simulink model "IEEE34bus_v2019b_Phasor_PI_ZIPload"  (R2024a)
settings: Solver=ode4  StartTime=0.0  StopTime=60  FixedStep=Ts  MaxStep=1e-4  RelTol=1e-4
InitFcn:
  | a=1; % Loading Factor
  | Ts=0.1;% For Delay Blocks in Voltage Regulator Controls
  | % phase to sequence conversion of RXB matrices
  | c=1*exp(sqrt(-1)*(120*pi/180));
  | T=[1 1 1;1 c*c c;1 c c*c];
  | Tinv=1/3*[1 1 1;1 c c*c;1 c*c c];
  | 
  | % Simulation data for the IEEE 34 Node Test Feeder model
  | mi2km = 1.60934;%  miles to km conversion
  | ft2km = 0.0003048; % feet to km conversion
  | ms2F = 1*1e-6/(2*pi*60);% microsiemens to Farads conversion
  | 
  | %% Configuration 300 - series reactance - ohm/mile
  | R_300 = [1.3368 0.2101 0.2130;0.2101 1.3238 0.2066;0.2130 0.2066 1.3294];
  | X_300 = [1.3343 0.5779 0.5015;0.5779 1.3569 0.4591;0.5015 0.4591 1.3471];
  | % charging susceptance - microsiemens/mile
  | B_300 = [5.3350 -1.5313 -0.9943;-1.5313 5.0979 -0.6212;-0.9943 -0.6212 4.8880];
  | 
  | R_300 = R_300/mi2km;
  | Rseq=Tinv*R_300*T;
  | R1_300=Rseq(2,2);R0_300=Rseq(1,1);
  | 
  | L_300 = (X_300/(2*pi*60))/mi2km;
  | Lseq=Tinv*L_300*T;
  | L1_300=Lseq(2,2);L0_300=Lseq(1,1);
  | 
  | C_300 =(B_300*ms2F)/mi2km;
  | Cseq=Tinv*C_300*T;
  | C1_300=Cseq(2,2);C0_300=Cseq(1,1);
  | 
  | %% Configuration 301 - series reactance - ohm/mile
  | R_301 = [1.9300 0.2327 0.2359;0.2327 1.9157 0.2288;0.2359 0.2288 1.9219];
  | X_301 = [1.4115 0.6442 0.5691;0.6442 1.4281 0.5238;0.5691 0.5238 1.4209];
  | % charging susceptance - microsiemens/mile
  | B_301 = [5.1207 -1.4364 -0.9402;-1.4364 4.9055 -0.5951;-0.9402 -0.5951 4.7154];
  | 
  | R_301 = R_301/mi2km;
  | Rseq=Tinv*R_301*T;
  | R1_301=Rseq(2,2);R0_301=Rseq(1,1);
  | 
  | L_301 = (X_301/(2*pi*60))/mi2km;
  | Lseq=Tinv*L_301*T;
  | L1_301=Lseq(2,2);L0_301=Lseq(1,1);
  | 
  | C_301 =(B_301*ms2F)/mi2km;
  | Cseq=Tinv*C_301*T;
  | C1_301=Cseq(2,2);C0_301=Cseq(1,1);
  | 
  | %% Configuration 302 - series reactance - ohm/mile
  | R_302 = [2.7995 0 0;0 0 0;0 0 0];
  | X_302 = [1.4855 0 0;0 0 0;0 0 0];
  | % charging susceptance - microsiemens/mile
  | B_302 = [4.2251 0 0;0 0 0;0 0 0];
  | 
  | R_302 = R_302/mi2km;
  | Rseq=Tinv*R_302*T;
  | R1_302=Rseq(2,2);R0_302=Rseq(1,1);
  | 
  | L_302 = (X_302/(2*pi*60))/mi2km;
  | Lseq=Tinv*L_302*T;
  | ... (+41 lines)
undefined symbols (not defined in the file or in its folder): find_system, j, m1, m2, m3, Rcc1, Rcc2, Rcc3
libraries: spsSeriesRLCBranchLib x160, spsGroundLib x106, spsVoltageMeasurementLib x100, spsControlledCurrentSourceLib x94, spsPowerPhasorLib x57, spsThreePhaseVIMeasurementLib x37, spsThreePhasePISectionLineLib x20, spsCurrentMeasurementLib x12, spsOnDelayLib x12, spsPiSectionLineLib x11, spsControlledVoltageSourceLib x6, spsDiscreteVariableTimeDelayLib x6
(part 3 of 8)

== system IEEE34bus_v2019b_Phasor_PI_ZIPload/834 D PQ ==
  Controlled Current Source : spsControlledCurrentSourceLib/Controlled Current Source  Initialize=off  Source_Type=AC  Amplitude=0  Phase=0  Frequency=0  Measurements=None
  Controlled Current Source1 : spsControlledCurrentSourceLib/Controlled Current Source  Initialize=off  Source_Type=AC  Amplitude=0  Phase=0  Frequency=0  Measurements=None
  Controlled Current Source2 : spsControlledCurrentSourceLib/Controlled Current Source  Initialize=off  Source_Type=AC  Amplitude=0  Phase=0  Frequency=0  Measurements=None
  Demux1 : Demux  Outputs=3
  Embedded MATLAB Function2 : MATLAB Function  TreatAsAtomicUnit=on
  Gain4 : Gain  Gain=sqrt(2)
  Gain5 : Gain  Gain=1/sqrt(2)
  Memory3 : Memory
  Mux5 : Mux  Inputs=3
  Rc+jXc1 : spsSeriesRLCBranchLib/Series RLC Branch  LConnTagsString=__new0  RConnTagsString=__new0  BranchType=R  Resistance=1e6  Inductance=1.6 / (120*pi) * 2  SetiL0=off  InitialCurrent=0  Capacitance=1e-6  Setx0=off  InitialVoltage=0  Measurements=None
  Rc+jXc2 : spsSeriesRLCBranchLib/Series RLC Branch  LConnTagsString=__new0  RConnTagsString=__new0  BranchType=R  Resistance=1e6  Inductance=1.6 / (120*pi) * 2  SetiL0=off  InitialCurrent=0  Capacitance=1e-6  Setx0=off  InitialVoltage=0  Measurements=None
  Rc+jXc3 : spsSeriesRLCBranchLib/Series RLC Branch  LConnTagsString=__new0  RConnTagsString=__new0  BranchType=R  Resistance=1e6  Inductance=1.6 / (120*pi) * 2  SetiL0=off  InitialCurrent=0  Capacitance=1e-6  Setx0=off  InitialVoltage=0  Measurements=None
  Voltage Measurement4 : spsVoltageMeasurementLib/Voltage Measurement  PhasorSimulation=on  OutputType=Complex  PSBequivalent=0
  Voltage Measurement5 : spsVoltageMeasurementLib/Voltage Measurement  PhasorSimulation=on  OutputType=Complex  PSBequivalent=0
  Voltage Measurement6 : spsVoltageMeasurementLib/Voltage Measurement  PhasorSimulation=on  OutputType=Complex  PSBequivalent=0
  " A" : PMIOPort  Tag=PMCPort  Side=Left
  " B" : PMIOPort  Tag=PMCPort  Port=2  Side=Left
  " C" : PMIOPort  Tag=PMCPort  Port=3  Side=Left
  wires:
  Embedded MATLAB Function2/1(Iinj) -> Gain4/1
  [vB] -> Mux5/2
  Voltage Measurement6/1 -> [vC]
  Mux5/1 -> Gain5/1
  [vA] -> Mux5/1
  Gain4/1 -> Memory3/1
  Gain5/1 -> Embedded MATLAB Function2/1(Vmeas)
  Demux1/1 -> Controlled Current Source/1
  Memory3/1 -> Demux1/1
  Demux1/2 -> Controlled Current Source1/1
  Voltage Measurement5/1 -> [vB]
  Demux1/3 -> Controlled Current Source2/1
  Voltage Measurement4/1 -> [vA]
  [vC] -> Mux5/3
  connections:
  Controlled Current Source2/LConn1 -- " C"/RConn1 -- Voltage Measurement6/LConn1 -- Rc+jXc3/LConn1 -- Voltage Measurement5/LConn2 -- Rc+jXc2/RConn1 -- Controlled Current Source1/RConn1
  " A"/RConn1 -- Voltage Measurement4/LConn1 -- Rc+jXc1/LConn1 -- Controlled Current Source/LConn1 -- Rc+jXc3/RConn1 -- Voltage Measurement6/LConn2 -- Controlled Current Source2/RConn1
  Rc+jXc1/RConn1 -- Controlled Current Source/RConn1 -- Voltage Measurement4/LConn2 -- " B"/RConn1 -- Voltage Measurement5/LConn1 -- Rc+jXc2/LConn1 -- Controlled Current Source1/LConn1

== system IEEE34bus_v2019b_Phasor_PI_ZIPload/834 D Z ==
  Controlled Current Source : spsControlledCurrentSourceLib/Controlled Current Source  Initialize=off  Source_Type=AC  Amplitude=0  Phase=0  Frequency=0  Measurements=None
  Controlled Current Source1 : spsControlledCurrentSourceLib/Controlled Current Source  Initialize=off  Source_Type=AC  Amplitude=0  Phase=0  Frequency=0  Measurements=None
  Controlled Current Source2 : spsControlledCurrentSourceLib/Controlled Current Source  Initialize=off  Source_Type=AC  Amplitude=0  Phase=0  Frequency=0  Measurements=None
  Demux1 : Demux  Outputs=3
  Embedded MATLAB Function2 : MATLAB Function  TreatAsAtomicUnit=on
  Gain4 : Gain  Gain=sqrt(2)
  Gain5 : Gain  Gain=1/sqrt(2)
  Memory3 : Memory
  Mux5 : Mux  Inputs=3
  Rc+jXc1 : spsSeriesRLCBranchLib/Series RLC Branch  LConnTagsString=__new0  RConnTagsString=__new0  BranchType=R  Resistance=1e6  Inductance=1.6 / (120*pi) * 2  SetiL0=off  InitialCurrent=0  Capacitance=1e-6  Setx0=off  InitialVoltage=0  Measurements=None
  Rc+jXc2 : spsSeriesRLCBranchLib/Series RLC Branch  LConnTagsString=__new0  RConnTagsString=__new0  BranchType=R  Resistance=1e6  Inductance=1.6 / (120*pi) * 2  SetiL0=off  InitialCurrent=0  Capacitance=1e-6  Setx0=off  InitialVoltage=0  Measurements=None
  Rc+jXc3 : spsSeriesRLCBranchLib/Series RLC Branch  LConnTagsString=__new0  RConnTagsString=__new0  BranchType=R  Resistance=1e6  Inductance=1.6 / (120*pi) * 2  SetiL0=off  InitialCurrent=0  Capacitance=1e-6  Setx0=off  InitialVoltage=0  Measurements=None
  Voltage Measurement4 : spsVoltageMeasurementLib/Voltage Measurement  PhasorSimulation=on  OutputType=Complex  PSBequivalent=0
  Voltage Measurement5 : spsVoltageMeasurementLib/Voltage Measurement  PhasorSimulation=on  OutputType=Complex  PSBequivalent=0
  Voltage Measurement6 : spsVoltageMeasurementLib/Voltage Measurement  PhasorSimulation=on  OutputType=Complex  PSBequivalent=0
  " A" : PMIOPort  Tag=PMCPort  Side=Left
  " B" : PMIOPort  Tag=PMCPort  Port=2  Side=Left
  " C" : PMIOPort  Tag=PMCPort  Port=3  Side=Left
  wires:
  [vC] -> Mux5/3
  Voltage Measurement4/1 -> [vA]
  Demux1/3 -> Controlled Current Source2/1
  Voltage Measurement5/1 -> [vB]
  Demux1/2 -> Controlled Current Source1/1
  Memory3/1 -> Demux1/1
  Demux1/1 -> Controlled Current Source/1
  Gain5/1 -> Embedded MATLAB Function2/1(Vmeas)
  Gain4/1 -> Memory3/1
  [vA] -> Mux5/1
  Mux5/1 -> Gain5/1
  Voltage Measurement6/1 -> [vC]
  [vB] -> Mux5/2
  Embedded MATLAB Function2/1(Iinj) -> Gain4/1
  connections:
  Controlled Current Source1/LConn1 -- Rc+jXc2/LConn1 -- Voltage Measurement5/LConn1 -- " B"/RConn1 -- Voltage Measurement4/LConn2 -- Controlled Current Source/RConn1 -- Rc+jXc1/RConn1
  Controlled Current Source2/RConn1 -- Voltage Measurement6/LConn2 -- Rc+jXc3/RConn1 -- Controlled Current Source/LConn1 -- Rc+jXc1/LConn1 -- Voltage Measurement4/LConn1 -- " A"/RConn1
  Controlled Current Source1/RConn1 -- Rc+jXc2/RConn1 -- Voltage Measurement5/LConn2 -- Rc+jXc3/LConn1 -- Voltage Measurement6/LConn1 -- " C"/RConn1 -- Controlled Current Source2/LConn1

== system IEEE34bus_v2019b_Phasor_PI_ZIPload/836 D I ==
  Controlled Current Source : spsControlledCurrentSourceLib/Controlled Current Source  Initialize=off  Source_Type=AC  Amplitude=0  Phase=0  Frequency=0  Measurements=None
  Controlled Current Source1 : spsControlledCurrentSourceLib/Controlled Current Source  Initialize=off  Source_Type=AC  Amplitude=0  Phase=0  Frequency=0  Measurements=None
  Controlled Current Source2 : spsControlledCurrentSourceLib/Controlled Current Source  Initialize=off  Source_Type=AC  Amplitude=0  Phase=0  Frequency=0  Measurements=None
  Demux1 : Demux  Outputs=3
  Embedded MATLAB Function2 : MATLAB Function  TreatAsAtomicUnit=on
  Gain4 : Gain  Gain=sqrt(2)
  Gain5 : Gain  Gain=1/sqrt(2)
  Memory3 : Memory
  Mux5 : Mux  Inputs=3
  Rc+jXc1 : spsSeriesRLCBranchLib/Series RLC Branch  LConnTagsString=__new0  RConnTagsString=__new0  BranchType=R  Resistance=1e6  Inductance=1.6 / (120*pi) * 2  SetiL0=off  InitialCurrent=0  Capacitance=1e-6  Setx0=off  InitialVoltage=0  Measurements=None
  Rc+jXc2 : spsSeriesRLCBranchLib/Series RLC Branch  LConnTagsString=__new0  RConnTagsString=__new0  BranchType=R  Resistance=1e6  Inductance=1.6 / (120*pi) * 2  SetiL0=off  InitialCurrent=0  Capacitance=1e-6  Setx0=off  InitialVoltage=0  Measurements=None
  Rc+jXc3 : spsSeriesRLCBranchLib/Series RLC Branch  LConnTagsString=__new0  RConnTagsString=__new0  BranchType=R  Resistance=1e6  Inductance=1.6 / (120*pi) * 2  SetiL0=off  InitialCurrent=0  Capacitance=1e-6  Setx0=off  InitialVoltage=0  Measurements=None
  Voltage Measurement4 : spsVoltageMeasurementLib/Voltage Measurement  PhasorSimulation=on  OutputType=Complex  PSBequivalent=0
  Voltage Measurement5 : spsVoltageMeasurementLib/Voltage Measurement  PhasorSimulation=on  OutputType=Complex  PSBequivalent=0
  Voltage Measurement6 : spsVoltageMeasurementLib/Voltage Measurement  PhasorSimulation=on  OutputType=Complex  PSBequivalent=0
  " A" : PMIOPort  Tag=PMCPort  Side=Left
  " B" : PMIOPort  Tag=PMCPort  Port=2  Side=Left
  " C" : PMIOPort  Tag=PMCPort  Port=3  Side=Left
  wires:
  Embedded MATLAB Function2/1(Iinj) -> Gain4/1
  [vB] -> Mux5/2
  Voltage Measurement6/1 -> [vC]
  Mux5/1 -> Gain5/1
  [vA] -> Mux5/1
  Gain4/1 -> Memory3/1
  Gain5/1 -> Embedded MATLAB Function2/1(Vmeas)
  Demux1/1 -> Controlled Current Source/1
  Memory3/1 -> Demux1/1
  Demux1/2 -> Controlled Current Source1/1
  Voltage Measurement5/1 -> [vB]
  Demux1/3 -> Controlled Current Source2/1
  Voltage Measurement4/1 -> [vA]
  [vC] -> Mux5/3
  connections:
  Controlled Current Source2/LConn1 -- " C"/RConn1 -- Voltage Measurement6/LConn1 -- Rc+jXc3/LConn1 -- Voltage Measurement5/LConn2 -- Rc+jXc2/RConn1 -- Controlled Current Source1/RConn1
  " A"/RConn1 -- Voltage Measurement4/LConn1 -- Rc+jXc1/LConn1 -- Controlled Current Source/LConn1 -- Rc+jXc3/RConn1 -- Voltage Measurement6/LConn2 -- Controlled Current Source2/RConn1
  Rc+jXc1/RConn1 -- Controlled Current Source/RConn1 -- Voltage Measurement4/LConn2 -- " B"/RConn1 -- Voltage Measurement5/LConn1 -- Rc+jXc2/LConn1 -- Controlled Current Source1/LConn1

== system IEEE34bus_v2019b_Phasor_PI_ZIPload/836 D PQ ==
  Controlled Current Source : spsControlledCurrentSourceLib/Controlled Current Source  Initialize=off  Source_Type=AC  Amplitude=0  Phase=0  Frequency=0  Measurements=None
  Controlled Current Source1 : spsControlledCurrentSourceLib/Controlled Current Source  Initialize=off  Source_Type=AC  Amplitude=0  Phase=0  Frequency=0  Measurements=None
  Controlled Current Source2 : spsControlledCurrentSourceLib/Controlled Current Source  Initialize=off  Source_Type=AC  Amplitude=0  Phase=0  Frequency=0  Measurements=None
  Demux1 : Demux  Outputs=3
  Embedded MATLAB Function2 : MATLAB Function  TreatAsAtomicUnit=on
  Gain4 : Gain  Gain=sqrt(2)
  Gain5 : Gain  Gain=1/sqrt(2)
  Memory3 : Memory
  Mux5 : Mux  Inputs=3
  Rc+jXc1 : spsSeriesRLCBranchLib/Series RLC Branch  LConnTagsString=__new0  RConnTagsString=__new0  BranchType=R  Resistance=1e6  Inductance=1.6 / (120*pi) * 2  SetiL0=off  InitialCurrent=0  Capacitance=1e-6  Setx0=off  InitialVoltage=0  Measurements=None
  Rc+jXc2 : spsSeriesRLCBranchLib/Series RLC Branch  LConnTagsString=__new0  RConnTagsString=__new0  BranchType=R  Resistance=1e6  Inductance=1.6 / (120*pi) * 2  SetiL0=off  InitialCurrent=0  Capacitance=1e-6  Setx0=off  InitialVoltage=0  Measurements=None
  Rc+jXc3 : spsSeriesRLCBranchLib/Series RLC Branch  LConnTagsString=__new0  RConnTagsString=__new0  BranchType=R  Resistance=1e6  Inductance=1.6 / (120*pi) * 2  SetiL0=off  InitialCurrent=0  Capacitance=1e-6  Setx0=off  InitialVoltage=0  Measurements=None
  Voltage Measurement4 : spsVoltageMeasurementLib/Voltage Measurement  PhasorSimulation=on  OutputType=Complex  PSBequivalent=0
  Voltage Measurement5 : spsVoltageMeasurementLib/Voltage Measurement  PhasorSimulation=on  OutputType=Complex  PSBequivalent=0
  Voltage Measurement6 : spsVoltageMeasurementLib/Voltage Measurement  PhasorSimulation=on  OutputType=Complex  PSBequivalent=0
  " A" : PMIOPort  Tag=PMCPort  Side=Left
  " B" : PMIOPort  Tag=PMCPort  Port=2  Side=Left
  " C" : PMIOPort  Tag=PMCPort  Port=3  Side=Left
  wires:
  Embedded MATLAB Function2/1(Iinj) -> Gain4/1
  [vB] -> Mux5/2
  Voltage Measurement6/1 -> [vC]
  Mux5/1 -> Gain5/1
  [vA] -> Mux5/1
  Gain4/1 -> Memory3/1
  Gain5/1 -> Embedded MATLAB Function2/1(Vmeas)
  Demux1/1 -> Controlled Current Source/1
  Memory3/1 -> Demux1/1
  Demux1/2 -> Controlled Current Source1/1
  Voltage Measurement5/1 -> [vB]
  Demux1/3 -> Controlled Current Source2/1
  Voltage Measurement4/1 -> [vA]
  [vC] -> Mux5/3
  connections:
  Controlled Current Source2/LConn1 -- " C"/RConn1 -- Voltage Measurement6/LConn1 -- Rc+jXc3/LConn1 -- Voltage Measurement5/LConn2 -- Rc+jXc2/RConn1 -- Controlled Current Source1/RConn1
  " A"/RConn1 -- Voltage Measurement4/LConn1 -- Rc+jXc1/LConn1 -- Controlled Current Source/LConn1 -- Rc+jXc3/RConn1 -- Voltage Measurement6/LConn2 -- Controlled Current Source2/RConn1
  Rc+jXc1/RConn1 -- Controlled Current Source/RConn1 -- Voltage Measurement4/LConn2 -- " B"/RConn1 -- Voltage Measurement5/LConn1 -- Rc+jXc2/LConn1 -- Controlled Current Source1/LConn1

== system IEEE34bus_v2019b_Phasor_PI_ZIPload/838 ==
  1 : spsThreePhaseVIMeasurementLib/Three-Phase V-I Measurement  VoltageMeasurement=phase-to-ground  SetLabelV=on  LabelV=V838  Vpu=off  VpuLL=off  CurrentMeasurement=no  SetLabelI=on  LabelI=I862  Ipu=off  Pbase=100e6  Vbase=24900  OutputType=Complex  PhasorSimulation=on  PSBequivalent=0
  Ground{1..2,9,12} (4 alike) : spsGroundLib/Ground  LConnTagsString=a
  b : PMIOPort  Side=Left
  B : PMIOPort  Port=2  Side=Right
  connections:
  1/LConn2 -- B/RConn1
  Ground12/LConn1 -- 1/LConn1
  b/RConn1 -- 1/RConn2
  Ground9/LConn1 -- 1/RConn1
  Ground2/LConn1 -- 1/LConn3
  Ground1/LConn1 -- 1/RConn3

== system IEEE34bus_v2019b_Phasor_PI_ZIPload/838 Y PQ ==
  Controlled Current Source : spsControlledCurrentSourceLib/Controlled Current Source  Initialize=off  Source_Type=AC  Amplitude=0  Phase=0  Frequency=0  Measurements=None
  Embedded MATLAB Function : MATLAB Function  TreatAsAtomicUnit=on
  Gain4 : Gain  Gain=sqrt(2)
  Gain5 : Gain  Gain=1/sqrt(2)
  Memory1 : Memory
  Rc+jXc1 : spsSeriesRLCBranchLib/Series RLC Branch  LConnTagsString=__new0  RConnTagsString=__new0  BranchType=R  Resistance=1e6  Inductance=1.6 / (120*pi) * 2  SetiL0=off  InitialCurrent=0  Capacitance=1e-6  Setx0=off  InitialVoltage=0  Measurements=None
  Voltage Measurement1 : spsVoltageMeasurementLib/Voltage Measurement  PhasorSimulation=on  OutputType=Complex  PSBequivalent=0
  " 2" : PMIOPort  Tag=PMCPort  Side=Left
  " 3" : PMIOPort  Tag=PMCPort  Port=2  Side=Right
  wires:
  Embedded MATLAB Function/1(Iinj) -> Gain4/1
  Memory1/1 -> Controlled Current Source/1
  Gain5/1 -> Embedded MATLAB Function/1(Vmeas)
  Voltage Measurement1/1 -> [v]
  [v] -> Gain5/1
  Gain4/1 -> Memory1/1
  connections:
  Controlled Current Source/RConn1 -- Rc+jXc1/RConn1 -- Voltage Measurement1/LConn2 -- " 3"/RConn1
  Rc+jXc1/LConn1 -- " 2"/RConn1 -- Voltage Measurement1/LConn1 -- Controlled Current Source/LConn1

== system IEEE34bus_v2019b_Phasor_PI_ZIPload/840 D I ==
  Controlled Current Source : spsControlledCurrentSourceLib/Controlled Current Source  Initialize=off  Source_Type=AC  Amplitude=0  Phase=0  Frequency=0  Measurements=None
  Controlled Current Source1 : spsControlledCurrentSourceLib/Controlled Current Source  Initialize=off  Source_Type=AC  Amplitude=0  Phase=0  Frequency=0  Measurements=None
  Controlled Current Source2 : spsControlledCurrentSourceLib/Controlled Current Source  Initialize=off  Source_Type=AC  Amplitude=0  Phase=0  Frequency=0  Measurements=None
  Demux1 : Demux  Outputs=3
  Embedded MATLAB Function2 : MATLAB Function  TreatAsAtomicUnit=on
  Gain4 : Gain  Gain=sqrt(2)
  Gain5 : Gain  Gain=1/sqrt(2)
  Memory3 : Memory
  Mux5 : Mux  Inputs=3
  Rc+jXc1 : spsSeriesRLCBranchLib/Series RLC Branch  LConnTagsString=__new0  RConnTagsString=__new0  BranchType=R  Resistance=1e6  Inductance=1.6 / (120*pi) * 2  SetiL0=off  InitialCurrent=0  Capacitance=1e-6  Setx0=off  InitialVoltage=0  Measurements=None
  Rc+jXc2 : spsSeriesRLCBranchLib/Series RLC Branch  LConnTagsString=__new0  RConnTagsString=__new0  BranchType=R  Resistance=1e6  Inductance=1.6 / (120*pi) * 2  SetiL0=off  InitialCurrent=0  Capacitance=1e-6  Setx0=off  InitialVoltage=0  Measurements=None
  Rc+jXc3 : spsSeriesRLCBranchLib/Series RLC Branch  LConnTagsString=__new0  RConnTagsString=__new0  BranchType=R  Resistance=1e6  Inductance=1.6 / (120*pi) * 2  SetiL0=off  InitialCurrent=0  Capacitance=1e-6  Setx0=off  InitialVoltage=0  Measurements=None
  Voltage Measurement4 : spsVoltageMeasurementLib/Voltage Measurement  PhasorSimulation=on  OutputType=Complex  PSBequivalent=0
  Voltage Measurement5 : spsVoltageMeasurementLib/Voltage Measurement  PhasorSimulation=on  OutputType=Complex  PSBequivalent=0
  Voltage Measurement6 : spsVoltageMeasurementLib/Voltage Measurement  PhasorSimulation=on  OutputType=Complex  PSBequivalent=0
  " A" : PMIOPort  Tag=PMCPort  Side=Left
  " B" : PMIOPort  Tag=PMCPort  Port=2  Side=Left
  " C" : PMIOPort  Tag=PMCPort  Port=3  Side=Left
  wires:
  [vC] -> Mux5/3
  Voltage Measurement4/1 -> [vA]
  Demux1/3 -> Controlled Current Source2/1
  Voltage Measurement5/1 -> [vB]
  Demux1/2 -> Controlled Current Source1/1
  Memory3/1 -> Demux1/1
  Demux1/1 -> Controlled Current Source/1
  Gain5/1 -> Embedded MATLAB Function2/1(Vmeas)
  Gain4/1 -> Memory3/1
  [vA] -> Mux5/1
  Mux5/1 -> Gain5/1
  Voltage Measurement6/1 -> [vC]
  [vB] -> Mux5/2
  Embedded MATLAB Function2/1(Iinj) -> Gain4/1
  connections:
  Controlled Current Source1/LConn1 -- Rc+jXc2/LConn1 -- Voltage Measurement5/LConn1 -- " B"/RConn1 -- Voltage Measurement4/LConn2 -- Controlled Current Source/RConn1 -- Rc+jXc1/RConn1
  Controlled Current Source2/RConn1 -- Voltage Measurement6/LConn2 -- Rc+jXc3/RConn1 -- Controlled Current Source/LConn1 -- Rc+jXc1/LConn1 -- Voltage Measurement4/LConn1 -- " A"/RConn1
  Controlled Current Source1/RConn1 -- Rc+jXc2/RConn1 -- Voltage Measurement5/LConn2 -- Rc+jXc3/LConn1 -- Voltage Measurement6/LConn1 -- " C"/RConn1 -- Controlled Current Source2/LConn1

== system IEEE34bus_v2019b_Phasor_PI_ZIPload/840 Y I ==
  Controlled Current Source : spsControlledCurrentSourceLib/Controlled Current Source  Initialize=off  Source_Type=AC  Amplitude=0  Phase=0  Frequency=0  Measurements=None
  Controlled Current Source1 : spsControlledCurrentSourceLib/Controlled Current Source  Initialize=off  Source_Type=AC  Amplitude=0  Phase=0  Frequency=0  Measurements=None
  Controlled Current Source2 : spsControlledCurrentSourceLib/Controlled Current Source  Initialize=off  Source_Type=AC  Amplitude=0  Phase=0  Frequency=0  Measurements=None
  Demux1 : Demux  Outputs=3
  Embedded MATLAB Function2 : MATLAB Function  TreatAsAtomicUnit=on
  Gain4 : Gain  Gain=sqrt(2)
  Gain5 : Gain  Gain=1/sqrt(2)
  Ground1 : spsGroundLib/Ground  LConnTagsString=a
  Memory3 : Memory
  Mux5 : Mux  Inputs=3
  Rc+jXc1 : spsSeriesRLCBranchLib/Series RLC Branch  LConnTagsString=__new0  RConnTagsString=__new0  BranchType=R  Resistance=1e6  Inductance=1.6 / (120*pi) * 2  SetiL0=off  InitialCurrent=0  Capacitance=1e-6  Setx0=off  InitialVoltage=0  Measurements=None
  Rc+jXc2 : spsSeriesRLCBranchLib/Series RLC Branch  LConnTagsString=__new0  RConnTagsString=__new0  BranchType=R  Resistance=1e6  Inductance=1.6 / (120*pi) * 2  SetiL0=off  InitialCurrent=0  Capacitance=1e-6  Setx0=off  InitialVoltage=0  Measurements=None
  Rc+jXc3 : spsSeriesRLCBranchLib/Series RLC Branch  LConnTagsString=__new0  RConnTagsString=__new0  BranchType=R  Resistance=1e6  Inductance=1.6 / (120*pi) * 2  SetiL0=off  InitialCurrent=0  Capacitance=1e-6  Setx0=off  InitialVoltage=0  Measurements=None
  Voltage Measurement4 : spsVoltageMeasurementLib/Voltage Measurement  PhasorSimulation=on  OutputType=Complex  PSBequivalent=0
  Voltage Measurement5 : spsVoltageMeasurementLib/Voltage Measurement  PhasorSimulation=on  OutputType=Complex  PSBequivalent=0
  Voltage Measurement6 : spsVoltageMeasurementLib/Voltage Measurement  PhasorSimulation=on  OutputType=Complex  PSBequivalent=0
  " A" : PMIOPort  Tag=PMCPort  Side=Left
  " B" : PMIOPort  Tag=PMCPort  Port=2  Side=Left
  " C" : PMIOPort  Tag=PMCPort  Port=3  Side=Left
  wires:
  Voltage Measurement4/1 -> [vA]
  Demux1/2 -> Controlled Current Source1/1
  Memory3/1 -> Demux1/1
  Demux1/1 -> Controlled Current Source/1
  Voltage Measurement6/1 -> [vC]
  Voltage Measurement5/1 -> [vB]
  Demux1/3 -> Controlled Current Source2/1
  Embedded MATLAB Function2/1(Iinj) -> Gain4/1
  Gain4/1 -> Memory3/1
  Mux5/1 -> Gain5/1
  Gain5/1 -> Embedded MATLAB Function2/1(Vmeas)
  [vA] -> Mux5/1
  [vB] -> Mux5/2
  [vC] -> Mux5/3
  connections:
  " B"/RConn1 -- Voltage Measurement5/LConn1 -- Rc+jXc2/LConn1 -- Controlled Current Source1/LConn1
  " A"/RConn1 -- Controlled Current Source/LConn1 -- Voltage Measurement4/LConn1 -- Rc+jXc1/LConn1
  Controlled Current Source2/LConn1 -- " C"/RConn1 -- Voltage Measurement6/LConn1 -- Rc+jXc3/LConn1
  Controlled Current Source1/RConn1 -- Rc+jXc2/RConn1 -- Voltage Measurement5/LConn2 -- Rc+jXc3/RConn1 -- Voltage Measurement6/LConn2 -- Controlled Current Source2/RConn1 -- Voltage Measurement4/LConn2 -- Rc+jXc1/RConn1 -- Controlled Current Source/RConn1 -- Ground1/LConn1

== system IEEE34bus_v2019b_Phasor_PI_ZIPload/842 Y PQ ==
  Controlled Current Source : spsControlledCurrentSourceLib/Controlled Current Source  Initialize=off  Source_Type=AC  Amplitude=0  Phase=0  Frequency=0  Measurements=None
  Embedded MATLAB Function : MATLAB Function  TreatAsAtomicUnit=on
  Gain4 : Gain  Gain=sqrt(2)
  Gain5 : Gain  Gain=1/sqrt(2)
  Memory1 : Memory
  Rc+jXc1 : spsSeriesRLCBranchLib/Series RLC Branch  LConnTagsString=__new0  RConnTagsString=__new0  BranchType=R  Resistance=1e6  Inductance=1.6 / (120*pi) * 2  SetiL0=off  InitialCurrent=0  Capacitance=1e-6  Setx0=off  InitialVoltage=0  Measurements=None
  Voltage Measurement1 : spsVoltageMeasurementLib/Voltage Measurement  PhasorSimulation=on  OutputType=Complex  PSBequivalent=0
  " 2" : PMIOPort  Tag=PMCPort  Side=Left
  " 3" : PMIOPort  Tag=PMCPort  Port=2  Side=Right
  wires:
  Embedded MATLAB Function/1(Iinj) -> Gain4/1
  Memory1/1 -> Controlled Current Source/1
  Gain5/1 -> Embedded MATLAB Function/1(Vmeas)
  Voltage Measurement1/1 -> [v]
  [v] -> Gain5/1
  Gain4/1 -> Memory1/1
  connections:
  Controlled Current Source/RConn1 -- Rc+jXc1/RConn1 -- Voltage Measurement1/LConn2 -- " 3"/RConn1
  Rc+jXc1/LConn1 -- " 2"/RConn1 -- Voltage Measurement1/LConn1 -- Controlled Current Source/LConn1

== system IEEE34bus_v2019b_Phasor_PI_ZIPload/844 Y PQ ==
  Controlled Current Source : spsControlledCurrentSourceLib/Controlled Current Source  Initialize=off  Source_Type=AC  Amplitude=0  Phase=0  Frequency=0  Measurements=None
  Embedded MATLAB Function : MATLAB Function  TreatAsAtomicUnit=on
  Gain4 : Gain  Gain=sqrt(2)
  Gain5 : Gain  Gain=1/sqrt(2)
  Memory1 : Memory
  Rc+jXc1 : spsSeriesRLCBranchLib/Series RLC Branch  LConnTagsString=__new0  RConnTagsString=__new0  BranchType=R  Resistance=1e6  Inductance=1.6 / (120*pi) * 2  SetiL0=off  InitialCurrent=0  Capacitance=1e-6  Setx0=off  InitialVoltage=0  Measurements=None
  Voltage Measurement1 : spsVoltageMeasurementLib/Voltage Measurement  PhasorSimulation=on  OutputType=Complex  PSBequivalent=0
  " 2" : PMIOPort  Tag=PMCPort  Side=Left
  " 3" : PMIOPort  Tag=PMCPort  Port=2  Side=Right
  wires:
  Gain4/1 -> Memory1/1
  [v] -> Gain5/1
  Voltage Measurement1/1 -> [v]
  Gain5/1 -> Embedded MATLAB Function/1(Vmeas)
  Memory1/1 -> Controlled Current Source/1
  Embedded MATLAB Function/1(Iinj) -> Gain4/1
  connections:
  Controlled Current Source/LConn1 -- Voltage Measurement1/LConn1 -- " 2"/RConn1 -- Rc+jXc1/LConn1
  " 3"/RConn1 -- Voltage Measurement1/LConn2 -- Rc+jXc1/RConn1 -- Controlled Current Source/RConn1

== system IEEE34bus_v2019b_Phasor_PI_ZIPload/844 Y PQ1 ==
  Controlled Current Source : spsControlledCurrentSourceLib/Controlled Current Source  Initialize=off  Source_Type=AC  Amplitude=0  Phase=0  Frequency=0  Measurements=None
  Controlled Current Source1 : spsControlledCurrentSourceLib/Controlled Current Source  Initialize=off  Source_Type=AC  Amplitude=0  Phase=0  Frequency=0  Measurements=None
  Controlled Current Source2 : spsControlledCurrentSourceLib/Controlled Current Source  Initialize=off  Source_Type=AC  Amplitude=0  Phase=0  Frequency=0  Measurements=None
  Demux1 : Demux  Outputs=3
  Embedded MATLAB Function2 : MATLAB Function  TreatAsAtomicUnit=on
  Gain4 : Gain  Gain=sqrt(2)
  Gain5 : Gain  Gain=1/sqrt(2)
  Ground1 : spsGroundLib/Ground  LConnTagsString=a
  Memory3 : Memory
  Mux5 : Mux  Inputs=3
  Rc+jXc1 : spsSeriesRLCBranchLib/Series RLC Branch  LConnTagsString=__new0  RConnTagsString=__new0  BranchType=R  Resistance=1e6  Inductance=1.6 / (120*pi) * 2  SetiL0=off  InitialCurrent=0  Capacitance=1e-6  Setx0=off  InitialVoltage=0  Measurements=None
  Rc+jXc2 : spsSeriesRLCBranchLib/Series RLC Branch  LConnTagsString=__new0  RConnTagsString=__new0  BranchType=R  Resistance=1e6  Inductance=1.6 / (120*pi) * 2  SetiL0=off  InitialCurrent=0  Capacitance=1e-6  Setx0=off  InitialVoltage=0  Measurements=None
  Rc+jXc3 : spsSeriesRLCBranchLib/Series RLC Branch  LConnTagsString=__new0  RConnTagsString=__new0  BranchType=R  Resistance=1e6  Inductance=1.6 / (120*pi) * 2  SetiL0=off  InitialCurrent=0  Capacitance=1e-6  Setx0=off  InitialVoltage=0  Measurements=None
  Voltage Measurement4 : spsVoltageMeasurementLib/Voltage Measurement  PhasorSimulation=on  OutputType=Complex  PSBequivalent=0
  Voltage Measurement5 : spsVoltageMeasurementLib/Voltage Measurement  PhasorSimulation=on  OutputType=Complex  PSBequivalent=0
  Voltage Measurement6 : spsVoltageMeasurementLib/Voltage Measurement  PhasorSimulation=on  OutputType=Complex  PSBequivalent=0
  " A" : PMIOPort  Tag=PMCPort  Side=Left
  " B" : PMIOPort  Tag=PMCPort  Port=2  Side=Left
  " C" : PMIOPort  Tag=PMCPort  Port=3  Side=Left
  wires:
  [vC] -> Mux5/3
  [vB] -> Mux5/2
  [vA] -> Mux5/1
  Gain5/1 -> Embedded MATLAB Function2/1(Vmeas)
  Mux5/1 -> Gain5/1
  Gain4/1 -> Memory3/1
  Embedded MATLAB Function2/1(Iinj) -> Gain4/1
  Demux1/3 -> Controlled Current Source2/1
  Voltage Measurement5/1 -> [vB]
  Voltage Measurement6/1 -> [vC]
  Demux1/1 -> Controlled Current Source/1
  Memory3/1 -> Demux1/1
  Demux1/2 -> Controlled Current Source1/1
  Voltage Measurement4/1 -> [vA]
  connections:
  Ground1/LConn1 -- Controlled Current Source/RConn1 -- Rc+jXc1/RConn1 -- Voltage Measurement4/LConn2 -- Controlled Current Source2/RConn1 -- Voltage Measurement6/LConn2 -- Rc+jXc3/RConn1 -- Voltage Measurement5/LConn2 -- Rc+jXc2/RConn1 -- Controlled Current Source1/RConn1
  Rc+jXc3/LConn1 -- Voltage Measurement6/LConn1 -- " C"/RConn1 -- Controlled Current Source2/LConn1
  Rc+jXc1/LConn1 -- Voltage Measurement4/LConn1 -- Controlled Current Source/LConn1 -- " A"/RConn1
  Controlled Current Source1/LConn1 -- Rc+jXc2/LConn1 -- Voltage Measurement5/LConn1 -- " B"/RConn1

== system IEEE34bus_v2019b_Phasor_PI_ZIPload/844 Y Z ==
  Controlled Current Source : spsControlledCurrentSourceLib/Controlled Current Source  Initialize=off  Source_Type=AC  Amplitude=0  Phase=0  Frequency=0  Measurements=None
  Controlled Current Source1 : spsControlledCurrentSourceLib/Controlled Current Source  Initialize=off  Source_Type=AC  Amplitude=0  Phase=0  Frequency=0  Measurements=None
  Controlled Current Source2 : spsControlledCurrentSourceLib/Controlled Current Source  Initialize=off  Source_Type=AC  Amplitude=0  Phase=0  Frequency=0  Measurements=None
  Demux1 : Demux  Outputs=3
  Embedded MATLAB Function2 : MATLAB Function  TreatAsAtomicUnit=on
  Gain4 : Gain  Gain=sqrt(2)
  Gain5 : Gain  Gain=1/sqrt(2)
  Ground1 : spsGroundLib/Ground  LConnTagsString=a
  Memory3 : Memory
  Mux5 : Mux  Inputs=3
  Rc+jXc1 : spsSeriesRLCBranchLib/Series RLC Branch  LConnTagsString=__new0  RConnTagsString=__new0  BranchType=R  Resistance=1e6  Inductance=1.6 / (120*pi) * 2  SetiL0=off  InitialCurrent=0  Capacitance=1e-6  Setx0=off  InitialVoltage=0  Measurements=None
  Rc+jXc2 : spsSeriesRLCBranchLib/Series RLC Branch  LConnTagsString=__new0  RConnTagsString=__new0  BranchType=R  Resistance=1e6  Inductance=1.6 / (120*pi) * 2  SetiL0=off  InitialCurrent=0  Capacitance=1e-6  Setx0=off  InitialVoltage=0  Measurements=None
  Rc+jXc3 : spsSeriesRLCBranchLib/Series RLC Branch  LConnTagsString=__new0  RConnTagsString=__new0  BranchType=R  Resistance=1e6  Inductance=1.6 / (120*pi) * 2  SetiL0=off  InitialCurrent=0  Capacitance=1e-6  Setx0=off  InitialVoltage=0  Measurements=None
  Voltage Measurement4 : spsVoltageMeasurementLib/Voltage Measurement  PhasorSimulation=on  OutputType=Complex  PSBequivalent=0
  Voltage Measurement5 : spsVoltageMeasurementLib/Voltage Measurement  PhasorSimulation=on  OutputType=Complex  PSBequivalent=0
  Voltage Measurement6 : spsVoltageMeasurementLib/Voltage Measurement  PhasorSimulation=on  OutputType=Complex  PSBequivalent=0
  " A" : PMIOPort  Tag=PMCPort  Side=Left
  " B" : PMIOPort  Tag=PMCPort  Port=2  Side=Left
  " C" : PMIOPort  Tag=PMCPort  Port=3  Side=Left
  wires:
  [vC] -> Mux5/3
  [vB] -> Mux5/2
  [vA] -> Mux5/1
  Gain5/1 -> Embedded MATLAB Function2/1(Vmeas)
  Mux5/1 -> Gain5/1
  Gain4/1 -> Memory3/1
  Embedded MATLAB Function2/1(Iinj) -> Gain4/1
  Demux1/3 -> Controlled Current Source2/1
  Voltage Measurement5/1 -> [vB]
  Voltage Measurement6/1 -> [vC]
  Demux1/1 -> Controlled Current Source/1
  Memory3/1 -> Demux1/1
  Demux1/2 -> Controlled Current Source1/1
  Voltage Measurement4/1 -> [vA]
  connections:
  Ground1/LConn1 -- Controlled Current Source/RConn1 -- Rc+jXc1/RConn1 -- Voltage Measurement4/LConn2 -- Controlled Current Source2/RConn1 -- Voltage Measurement6/LConn2 -- Rc+jXc3/RConn1 -- Voltage Measurement5/LConn2 -- Rc+jXc2/RConn1 -- Controlled Current Source1/RConn1
  Rc+jXc3/LConn1 -- Voltage Measurement6/LConn1 -- " C"/RConn1 -- Controlled Current Source2/LConn1
  Rc+jXc1/LConn1 -- Voltage Measurement4/LConn1 -- Controlled Current Source/LConn1 -- " A"/RConn1
  Controlled Current Source1/LConn1 -- Rc+jXc2/LConn1 -- Voltage Measurement5/LConn1 -- " B"/RConn1

== system IEEE34bus_v2019b_Phasor_PI_ZIPload/846 Y PQ ==
  Controlled Current Source : spsControlledCurrentSourceLib/Controlled Current Source  Initialize=off  Source_Type=AC  Amplitude=0  Phase=0  Frequency=0  Measurements=None
  Controlled Current Source1 : spsControlledCurrentSourceLib/Controlled Current Source  Initialize=off  Source_Type=AC  Amplitude=0  Phase=0  Frequency=0  Measurements=None
  Controlled Current Source2 : spsControlledCurrentSourceLib/Controlled Current Source  Initialize=off  Source_Type=AC  Amplitude=0  Phase=0  Frequency=0  Measurements=None
  Demux1 : Demux  Outputs=3
  Embedded MATLAB Function2 : MATLAB Function  TreatAsAtomicUnit=on
  Gain4 : Gain  Gain=sqrt(2)
  Gain5 : Gain  Gain=1/sqrt(2)
  Ground1 : spsGroundLib/Ground  LConnTagsString=a
  Memory3 : Memory
  Mux5 : Mux  Inputs=3
  Rc+jXc1 : spsSeriesRLCBranchLib/Series RLC Branch  LConnTagsString=__new0  RConnTagsString=__new0  BranchType=R  Resistance=1e6  Inductance=1.6 / (120*pi) * 2  SetiL0=off  InitialCurrent=0  Capacitance=1e-6  Setx0=off  InitialVoltage=0  Measurements=None
  Rc+jXc2 : spsSeriesRLCBranchLib/Series RLC Branch  LConnTagsString=__new0  RConnTagsString=__new0  BranchType=R  Resistance=1e6  Inductance=1.6 / (120*pi) * 2  SetiL0=off  InitialCurrent=0  Capacitance=1e-6  Setx0=off  InitialVoltage=0  Measurements=None
  Rc+jXc3 : spsSeriesRLCBranchLib/Series RLC Branch  LConnTagsString=__new0  RConnTagsString=__new0  BranchType=R  Resistance=1e6  Inductance=1.6 / (120*pi) * 2  SetiL0=off  InitialCurrent=0  Capacitance=1e-6  Setx0=off  InitialVoltage=0  Measurements=None
  Voltage Measurement4 : spsVoltageMeasurementLib/Voltage Measurement  PhasorSimulation=on  OutputType=Complex  PSBequivalent=0
  Voltage Measurement5 : spsVoltageMeasurementLib/Voltage Measurement  PhasorSimulation=on  OutputType=Complex  PSBequivalent=0
  Voltage Measurement6 : spsVoltageMeasurementLib/Voltage Measurement  PhasorSimulation=on  OutputType=Complex  PSBequivalent=0
  " A" : PMIOPort  Tag=PMCPort  Side=Left
  " B" : PMIOPort  Tag=PMCPort  Port=2  Side=Left
  " C" : PMIOPort  Tag=PMCPort  Port=3  Side=Left
  wires:
  Voltage Measurement4/1 -> [vA]
  Demux1/2 -> Controlled Current Source1/1
  Memory3/1 -> Demux1/1
  Demux1/1 -> Controlled Current Source/1
  Voltage Measurement6/1 -> [vC]
  Voltage Measurement5/1 -> [vB]
  Demux1/3 -> Controlled Current Source2/1
  Embedded MATLAB Function2/1(Iinj) -> Gain4/1
  Gain4/1 -> Memory3/1
  Mux5/1 -> Gain5/1
  Gain5/1 -> Embedded MATLAB Function2/1(Vmeas)
  [vA] -> Mux5/1
  [vB] -> Mux5/2
  [vC] -> Mux5/3
  connections:
  " B"/RConn1 -- Voltage Measurement5/LConn1 -- Rc+jXc2/LConn1 -- Controlled Current Source1/LConn1
  " A"/RConn1 -- Controlled Current Source/LConn1 -- Voltage Measurement4/LConn1 -- Rc+jXc1/LConn1
  Controlled Current Source2/LConn1 -- " C"/RConn1 -- Voltage Measurement6/LConn1 -- Rc+jXc3/LConn1
  Controlled Current Source1/RConn1 -- Rc+jXc2/RConn1 -- Voltage Measurement5/LConn2 -- Rc+jXc3/RConn1 -- Voltage Measurement6/LConn2 -- Controlled Current Source2/RConn1 -- Voltage Measurement4/LConn2 -- Rc+jXc1/RConn1 -- Controlled Current Source/RConn1 -- Ground1/LConn1

== system IEEE34bus_v2019b_Phasor_PI_ZIPload/846 Y PQ1 ==
  Controlled Current Source : spsControlledCurrentSourceLib/Controlled Current Source  Initialize=off  Source_Type=AC  Amplitude=0  Phase=0  Frequency=0  Measurements=None
  Embedded MATLAB Function : MATLAB Function  TreatAsAtomicUnit=on
  Gain4 : Gain  Gain=sqrt(2)
  Gain5 : Gain  Gain=1/sqrt(2)
  Memory1 : Memory
  Rc+jXc1 : spsSeriesRLCBranchLib/Series RLC Branch  LConnTagsString=__new0  RConnTagsString=__new0  BranchType=R  Resistance=1e6  Inductance=1.6 / (120*pi) * 2  SetiL0=off  InitialCurrent=0  Capacitance=1e-6  Setx0=off  InitialVoltage=0  Measurements=None
  Voltage Measurement1 : spsVoltageMeasurementLib/Voltage Measurement  PhasorSimulation=on  OutputType=Complex  PSBequivalent=0
  " 2" : PMIOPort  Tag=PMCPort  Side=Left
  " 3" : PMIOPort  Tag=PMCPort  Port=2  Side=Right
  wires:
  Gain4/1 -> Memory1/1
  [v] -> Gain5/1
  Voltage Measurement1/1 -> [v]
  Gain5/1 -> Embedded MATLAB Function/1(Vmeas)
  Memory1/1 -> Controlled Current Source/1
  Embedded MATLAB Function/1(Iinj) -> Gain4/1
  connections:
  Controlled Current Source/LConn1 -- Voltage Measurement1/LConn1 -- " 2"/RConn1 -- Rc+jXc1/LConn1
  " 3"/RConn1 -- Voltage Measurement1/LConn2 -- Rc+jXc1/RConn1 -- Controlled Current Source/RConn1

== system IEEE34bus_v2019b_Phasor_PI_ZIPload/848 D PQ ==
  Controlled Current Source : spsControlledCurrentSourceLib/Controlled Current Source  Initialize=off  Source_Type=AC  Amplitude=0  Phase=0  Frequency=0  Measurements=None
  Controlled Current Source1 : spsControlledCurrentSourceLib/Controlled Current Source  Initialize=off  Source_Type=AC  Amplitude=0  Phase=0  Frequency=0  Measurements=None
  Controlled Current Source2 : spsControlledCurrentSourceLib/Controlled Current Source  Initialize=off  Source_Type=AC  Amplitude=0  Phase=0  Frequency=0  Measurements=None
  Demux1 : Demux  Outputs=3
  Embedded MATLAB Function2 : MATLAB Function  TreatAsAtomicUnit=on
  Gain4 : Gain  Gain=sqrt(2)
  Gain5 : Gain  Gain=1/sqrt(2)
  Memory3 : Memory
  Mux5 : Mux  Inputs=3
  Rc+jXc1 : spsSeriesRLCBranchLib/Series RLC Branch  LConnTagsString=__new0  RConnTagsString=__new0  BranchType=R  Resistance=1e6  Inductance=1.6 / (120*pi) * 2  SetiL0=off  InitialCurrent=0  Capacitance=1e-6  Setx0=off  InitialVoltage=0  Measurements=None
  Rc+jXc2 : spsSeriesRLCBranchLib/Series RLC Branch  LConnTagsString=__new0  RConnTagsString=__new0  BranchType=R  Resistance=1e6  Inductance=1.6 / (120*pi) * 2  SetiL0=off  InitialCurrent=0  Capacitance=1e-6  Setx0=off  InitialVoltage=0  Measurements=None
  Rc+jXc3 : spsSeriesRLCBranchLib/Series RLC Branch  LConnTagsString=__new0  RConnTagsString=__new0  BranchType=R  Resistance=1e6  Inductance=1.6 / (120*pi) * 2  SetiL0=off  InitialCurrent=0  Capacitance=1e-6  Setx0=off  InitialVoltage=0  Measurements=None
  Voltage Measurement4 : spsVoltageMeasurementLib/Voltage Measurement  PhasorSimulation=on  OutputType=Complex  PSBequivalent=0
  Voltage Measurement5 : spsVoltageMeasurementLib/Voltage Measurement  PhasorSimulation=on  OutputType=Complex  PSBequivalent=0
  Voltage Measurement6 : spsVoltageMeasurementLib/Voltage Measurement  PhasorSimulation=on  OutputType=Complex  PSBequivalent=0
  " A" : PMIOPort  Tag=PMCPort  Side=Left
  " B" : PMIOPort  Tag=PMCPort  Port=2  Side=Left
  " C" : PMIOPort  Tag=PMCPort  Port=3  Side=Left
  wires:
  [vC] -> Mux5/3
  Voltage Measurement4/1 -> [vA]
  Demux1/3 -> Controlled Current Source2/1
  Voltage Measurement5/1 -> [vB]
  Demux1/2 -> Controlled Current Source1/1
  Memory3/1 -> Demux1/1
  Demux1/1 -> Controlled Current Source/1
  Gain5/1 -> Embedded MATLAB Function2/1(Vmeas)
  Gain4/1 -> Memory3/1
  [vA] -> Mux5/1
  Mux5/1 -> Gain5/1
  Voltage Measurement6/1 -> [vC]
  [vB] -> Mux5/2
  Embedded MATLAB Function2/1(Iinj) -> Gain4/1
  connections:
  Controlled Current Source1/LConn1 -- Rc+jXc2/LConn1 -- Voltage Measurement5/LConn1 -- " B"/RConn1 -- Voltage Measurement4/LConn2 -- Controlled Current Source/RConn1 -- Rc+jXc1/RConn1
  Controlled Current Source2/RConn1 -- Voltage Measurement6/LConn2 -- Rc+jXc3/RConn1 -- Controlled Current Source/LConn1 -- Rc+jXc1/LConn1 -- Voltage Measurement4/LConn1 -- " A"/RConn1
  Controlled Current Source1/RConn1 -- Rc+jXc2/RConn1 -- Voltage Measurement5/LConn2 -- Rc+jXc3/LConn1 -- Voltage Measurement6/LConn1 -- " C"/RConn1 -- Controlled Current Source2/LConn1

== system IEEE34bus_v2019b_Phasor_PI_ZIPload/848 Y PQ ==
  Controlled Current Source : spsControlledCurrentSourceLib/Controlled Current Source  Initialize=off  Source_Type=AC  Amplitude=0  Phase=0  Frequency=0  Measurements=None
  Embedded MATLAB Function : MATLAB Function  TreatAsAtomicUnit=on
  Gain4 : Gain  Gain=sqrt(2)
  Gain5 : Gain  Gain=1/sqrt(2)
  Memory1 : Memory
  Rc+jXc1 : spsSeriesRLCBranchLib/Series RLC Branch  LConnTagsString=__new0  RConnTagsString=__new0  BranchType=R  Resistance=1e6  Inductance=1.6 / (120*pi) * 2  SetiL0=off  InitialCurrent=0  Capacitance=1e-6  Setx0=off  InitialVoltage=0  Measurements=None
  Voltage Measurement1 : spsVoltageMeasurementLib/Voltage Measurement  PhasorSimulation=on  OutputType=Complex  PSBequivalent=0
  " 2" : PMIOPort  Tag=PMCPort  Side=Left
  " 3" : PMIOPort  Tag=PMCPort  Port=2  Side=Right
  wires:
  Embedded MATLAB Function/1(Iinj) -> Gain4/1
  Memory1/1 -> Controlled Current Source/1
  Gain5/1 -> Embedded MATLAB Function/1(Vmeas)
  Voltage Measurement1/1 -> [v]
  [v] -> Gain5/1
  Gain4/1 -> Memory1/1
  connections:
  Controlled Current Source/RConn1 -- Rc+jXc1/RConn1 -- Voltage Measurement1/LConn2 -- " 3"/RConn1
  Rc+jXc1/LConn1 -- " 2"/RConn1 -- Voltage Measurement1/LConn1 -- Controlled Current Source/LConn1

== system IEEE34bus_v2019b_Phasor_PI_ZIPload/852-832 301 ==
  Config300 : spsMutualInductanceLib/Mutual Inductance  LConnTagsString=a|b|c  RConnTagsString=A|B|C  TypeOfMutual=Generalized mutual inductance  NumberOfWindings=3  SelfImpedance1=[1.1 1.1e-03]  SelfImpedance2=[ 1.1 1.1e-03]  ThreeWindings=on  SelfImpedance3=[ 1.1 1.1e-03]  MutualImpedance=[1.0 1.0e-03]  InductanceMatrix=Ll* L  ResistanceMatrix=Rl* L  Measurements=None
      settings: LibrarySourceBlock=sps_lib/Passives/Mutual Inductance
  Ground{1..6} (6 alike) : spsGroundLib/Ground  LConnTagsString=a
  Series RLC Branch : spsSeriesRLCBranchLib/Series RLC Branch  LConnTagsString=__new0  RConnTagsString=__new0  BranchType=C  Resistance=1  Inductance=1e-3  SetiL0=off  InitialCurrent=0  Capacitance=Cl(1,3)/2*L  Setx0=off  InitialVoltage=0  Measurements=None
  Series RLC Branch1 : spsSeriesRLCBranchLib/Series RLC Branch  LConnTagsString=__new0  RConnTagsString=__new0  BranchType=C  Resistance=1  Inductance=1e-3  SetiL0=off  InitialCurrent=0  Capacitance=Cl(1,3)/2*L  Setx0=off  InitialVoltage=0  Measurements=None
  Series RLC Branch10 : spsSeriesRLCBranchLib/Series RLC Branch  LConnTagsString=__new0  RConnTagsString=__new0  BranchType=C  Resistance=1  Inductance=1e-3  SetiL0=off  InitialCurrent=0  Capacitance=Cl(2,2)/2*L  Setx0=off  InitialVoltage=0  Measurements=None
  Series RLC Branch11 : spsSeriesRLCBranchLib/Series RLC Branch  LConnTagsString=__new0  RConnTagsString=__new0  BranchType=C  Resistance=1  Inductance=1e-3  SetiL0=off  InitialCurrent=0  Capacitance=Cl(1,1)/2*L  Setx0=off  InitialVoltage=0  Measurements=None
  Series RLC Branch2 : spsSeriesRLCBranchLib/Series RLC Branch  LConnTagsString=__new0  RConnTagsString=__new0  BranchType=C  Resistance=1  Inductance=1e-3  SetiL0=off  InitialCurrent=0  Capacitance=Cl(1,2)/2*L  Setx0=off  InitialVoltage=0  Measurements=None
  Series RLC Branch3 : spsSeriesRLCBranchLib/Series RLC Branch  LConnTagsString=__new0  RConnTagsString=__new0  BranchType=C  Resistance=1  Inductance=1e-3  SetiL0=off  InitialCurrent=0  Capacitance=Cl(2,3)/2*L  Setx0=off  InitialVoltage=0  Measurements=None
  Series RLC Branch4 : spsSeriesRLCBranchLib/Series RLC Branch  LConnTagsString=__new0  RConnTagsString=__new0  BranchType=C  Resistance=1  Inductance=1e-3  SetiL0=off  InitialCurrent=0  Capacitance=Cl(1,2)/2*L  Setx0=off  InitialVoltage=0  Measurements=None
  Series RLC Branch5 : spsSeriesRLCBranchLib/Series RLC Branch  LConnTagsString=__new0  RConnTagsString=__new0  BranchType=C  Resistance=1  Inductance=1e-3  SetiL0=off  InitialCurrent=0  Capacitance=Cl(2,3)/2*L  Setx0=off  InitialVoltage=0  Measurements=None
  Series RLC Branch6 : spsSeriesRLCBranchLib/Series RLC Branch  LConnTagsString=__new0  RConnTagsString=__new0  BranchType=C  Resistance=1  Inductance=1e-3  SetiL0=off  InitialCurrent=0  Capacitance=Cl(1,1)/2*L  Setx0=off  InitialVoltage=0  Measurements=None
  Series RLC Branch7 : spsSeriesRLCBranchLib/Series RLC Branch  LConnTagsString=__new0  RConnTagsString=__new0  BranchType=C  Resistance=1  Inductance=1e-3  SetiL0=off  InitialCurrent=0  Capacitance=Cl(2,2)/2*L  Setx0=off  InitialVoltage=0  Measurements=None
  Series RLC Branch8 : spsSeriesRLCBranchLib/Series RLC Branch  LConnTagsString=__new0  RConnTagsString=__new0  BranchType=C  Resistance=1  Inductance=1e-3  SetiL0=off  InitialCurrent=0  Capacitance=Cl(3,3)/2*L  Setx0=off  InitialVoltage=0  Measurements=None
  Series RLC Branch9 : spsSeriesRLCBranchLib/Series RLC Branch  LConnTagsString=__new0  RConnTagsString=__new0  BranchType=C  Resistance=1  Inductance=1e-3  SetiL0=off  InitialCurrent=0  Capacitance=Cl(3,3)/2*L  Setx0=off  InitialVoltage=0  Measurements=None
  A In : PMIOPort  Side=Left
  B In : PMIOPort  Port=2  Side=Left
  C in : PMIOPort  Port=3  Side=Left
  A Out : PMIOPort  Port=4  Side=Right
  B Out : PMIOPort  Port=5  Side=Right
  C Out : PMIOPort  Port=6  Side=Right
  connections:
  Series RLC Branch6/RConn1 -- Ground2/LConn1
  Series RLC Branch7/RConn1 -- Ground4/LConn1
  Series RLC Branch8/RConn1 -- Ground5/LConn1
  Ground6/LConn1 -- Series RLC Branch9/RConn1
  Ground1/LConn1 -- Series RLC Branch10/RConn1
  Ground3/LConn1 -- Series RLC Branch11/RConn1
  C Out/RConn1 -- Series RLC Branch1/RConn1 -- Series RLC Branch3/RConn1 -- Series RLC Branch8/LConn1 -- Config300/RConn3
  C in/RConn1 -- Series RLC Branch/RConn1 -- Series RLC Branch5/RConn1 -- Series RLC Branch9/LConn1 -- Config300/LConn3
  A Out/RConn1 -- Series RLC Branch1/LConn1 -- Series RLC Branch2/LConn1 -- Series RLC Branch6/LConn1 -- Config300/RConn1
  A In/RConn1 -- Series RLC Branch/LConn1 -- Series RLC Branch4/LConn1 -- Series RLC Branch11/LConn1 -- Config300/LConn1
  B Out/RConn1 -- Series RLC Branch2/RConn1 -- Series RLC Branch3/LConn1 -- Series RLC Branch7/LConn1 -- Config300/RConn2
  B In/RConn1 -- Config300/LConn2 -- Series RLC Branch10/LConn1 -- Series RLC Branch5/LConn1 -- Series RLC Branch4/RConn1

== system IEEE34bus_v2019b_Phasor_PI_ZIPload/854 Y PQ ==
  Controlled Current Source : spsControlledCurrentSourceLib/Controlled Current Source  Initialize=off  Source_Type=AC  Amplitude=0  Phase=0  Frequency=0  Measurements=None
  Embedded MATLAB Function : MATLAB Function  TreatAsAtomicUnit=on
  Gain4 : Gain  Gain=sqrt(2)
  Gain5 : Gain  Gain=1/sqrt(2)
  Memory1 : Memory
  Rc+jXc1 : spsSeriesRLCBranchLib/Series RLC Branch  LConnTagsString=__new0  RConnTagsString=__new0  BranchType=R  Resistance=1e6  Inductance=1.6 / (120*pi) * 2  SetiL0=off  InitialCurrent=0  Capacitance=1e-6  Setx0=off  InitialVoltage=0  Measurements=None
  Voltage Measurement1 : spsVoltageMeasurementLib/Voltage Measurement  PhasorSimulation=on  OutputType=Complex  PSBequivalent=0
  " 2" : PMIOPort  Tag=PMCPort  Side=Left
  " 3" : PMIOPort  Tag=PMCPort  Port=2  Side=Right
  wires:
  Embedded MATLAB Function/1(Iinj) -> Gain4/1
  Memory1/1 -> Controlled Current Source/1
  Gain5/1 -> Embedded MATLAB Function/1(Vmeas)
  Voltage Measurement1/1 -> [v]
  [v] -> Gain5/1
  Gain4/1 -> Memory1/1
  connections:
  Controlled Current Source/RConn1 -- Rc+jXc1/RConn1 -- Voltage Measurement1/LConn2 -- " 3"/RConn1
  Rc+jXc1/LConn1 -- " 2"/RConn1 -- Voltage Measurement1/LConn1 -- Controlled Current Source/LConn1
